simulink model "SatelliteAttitudeTargeting"  (R2020b)
settings: Solver=VariableStepAuto  StartTime=0.0  StopTime=30  MinStep=5e-5  RelTol=2.8421709430404007E-14
values from neighbouring files (symbols this model uses):
  dt_delay = 0.01    [main.m]
  hwdotmax = 0.004    [controlDesign.m]
  hwmax = 0.015    [controlDesign.m]
  Kd = diag([Kd1; Kd2; Kd3])    [controlDesign.m]
  Ko = 3075    [controlDesign.m]
  Kp = 8.0    (= 8)    [controlDesign.m]
  Po = 400    [controlDesign.m]
  s = tf('s')    [controlDesign.m]
  safety = 0.5    [controlDesign.m]
  wn = 2*pi*10    (= 62.8318530718)    [controlDesign.m]
  zeta = sqrt(2)/2    [controlDesign.m]
  Zo = 0.01    [controlDesign.m]
undefined symbols (not defined in the file or in its folder): A_BP, A_PB, J_C_B, J_C_P, md, ms, q_PB, rcb_B, rlb_B, X, Y, Z
libraries: sm_lib x10, nesl_utility x4
settings Model: Creator=bbingham  LastModifiedBy=tjones
settings SolverCC: MaxConsecutiveMinStep=2
settings DataIOCC: SaveOutput=off  SignalLogging=off  DSMLogging=off  ReturnWorkspaceOutputs=off
settings DebuggingCC: ArithmeticOperatorsInVariantConditions=warning
settings SFSimCC: SimUseLocalCustomCode=off  CustomCodeUndefinedFunction=UseInterfaceOnly
settings RTWCC: Description=Simulink Desktop Real-Time  SystemTargetFile=sldrt.tlc  TemplateMakefile=sldrt.tmf  RTWUseLocalCustomCode=off  RTWCompilerOptimization=on
settings CodeAppCC: MaxIdLength=95  StateflowObjectComments=on
settings TargetCC: TargetPreCompLibLocation=C:\Program Files\MATLAB\R2020a\toolbox\sldrt\lib\win64  TargetLangStandard=C99 (ISO)  SupportVariableSizeSignals=on
settings SimscapeCC: SimscapeNormalizeSystem=off

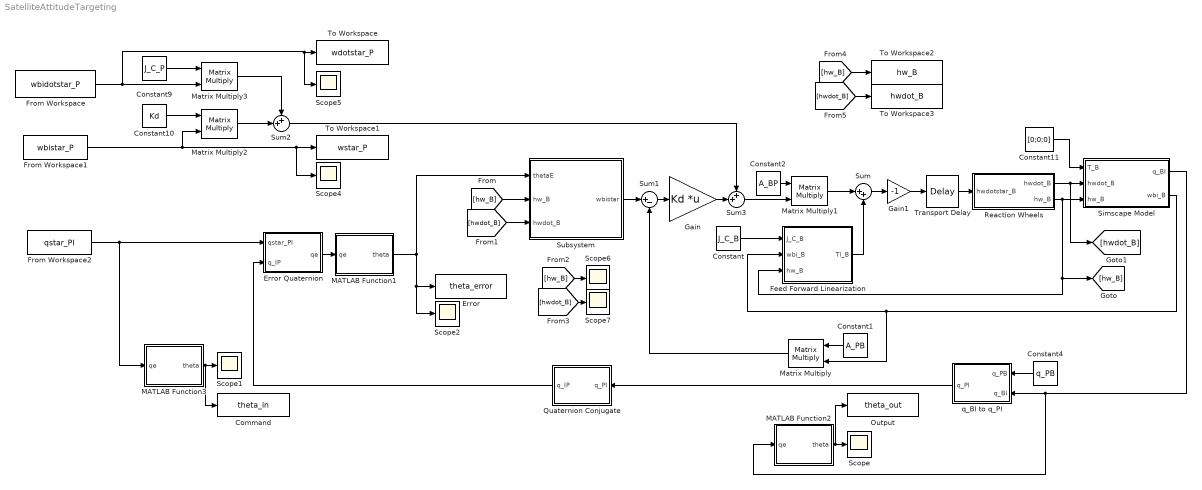
== system SatelliteAttitudeTargeting ==
  Command : ToWorkspace  VariableName=theta_in  SaveFormat=Timeseries  SampleTime=-1
  Constant : Constant  Value=J_C_B
  Constant1 : Constant  Value=A_PB
  Constant10 : Constant  Value=Kd
  Constant11 : Constant  Value=[0;0;0]
  Constant2 : Constant  Value=A_BP
  Constant4 : Constant  Value=q_PB  OutDataTypeStr=Bus: qBus
  Constant9 : Constant  Value=J_C_P
  Error : ToWorkspace  VariableName=theta_error  SaveFormat=Timeseries  SampleTime=-1
  Error Quaternion : MATLAB Function  TreatAsAtomicUnit=on
  Feed Forward Linearization : MATLAB Function  TreatAsAtomicUnit=on
  From Workspace : FromWorkspace  VariableName=wbidotstar_P
  From Workspace1 : FromWorkspace  VariableName=wbistar_P
  From Workspace2 : FromWorkspace  VariableName=qstar_PI  OutDataTypeStr=Bus: qBus
  Gain : Gain  Gain=Kd  Multiplication=Matrix(K*u) (u vector)
  Gain1 : Gain  Gain=-1
  MATLAB Function1 : MATLAB Function  TreatAsAtomicUnit=on
  MATLAB Function2 : MATLAB Function  TreatAsAtomicUnit=on
  MATLAB Function3 : MATLAB Function  TreatAsAtomicUnit=on
  Matrix Multiply{,1..3} (4 alike) : Product  Multiplication=Matrix(*)
  Output : ToWorkspace  VariableName=theta_out  SaveFormat=Timeseries  SampleTime=-1
  Quaternion Conjugate : MATLAB Function  TreatAsAtomicUnit=on
  Reaction Wheels : Subsystem
  Scope{,1..2,4..7} (7 alike) : Scope
  Simscape Model : Subsystem  TreatAsAtomicUnit=on
  Subsystem : Subsystem
  Sum : Sum  Inputs=|++
  Sum1 : Sum  Inputs=|+-
  Sum2 : Sum  Inputs=++|
  Sum3 : Sum  Inputs=++|
  To Workspace : ToWorkspace  VariableName=wdotstar_P  SaveFormat=Timeseries  SampleTime=-1
  To Workspace1 : ToWorkspace  VariableName=wstar_P  SaveFormat=Timeseries  SampleTime=-1
  To Workspace2 : ToWorkspace  VariableName=hw_B  SaveFormat=Timeseries  SampleTime=-1
  To Workspace3 : ToWorkspace  VariableName=hwdot_B  SaveFormat=Timeseries  SampleTime=-1
  Transport Delay : TransportDelay  DelayTime=dt_delay  BufferSize=3072
  q_BI to q_PI : MATLAB Function  TreatAsAtomicUnit=on
  wires:
  Simscape Model/2(wbi_B) -> Matrix Multiply/2, Feed Forward Linearization/2(wbi_B)
  Feed Forward Linearization/1(Tl_B) -> Sum/2
  Constant/1 -> Feed Forward Linearization/1(J_C_B)
  Constant1/1 -> Matrix Multiply/1
  Matrix Multiply/1 -> Sum1/2
  Sum1/1 -> Gain/1
  Constant2/1 -> Matrix Multiply1/1
  Matrix Multiply1/1 -> Sum/1
  Constant4/1 -> q_BI to q_PI/1(q_PB)
  Simscape Model/1(q_BI) -> MATLAB Function2/1(qe), q_BI to q_PI/2(q_BI)
  q_BI to q_PI/1(q_PI) -> Quaternion Conjugate/1(q_PI)
  Error Quaternion/1(qe) -> MATLAB Function1/1(qe)
  From Workspace2/1 -> Error Quaternion/1(qstar_PI), MATLAB Function3/1(qe)
  Quaternion Conjugate/1(q_IP) -> Error Quaternion/2(q_IP)
  MATLAB Function1/1(theta) -> Subsystem/1(thetaE), Error/1, Scope2/1
  MATLAB Function2/1(theta) -> Output/1, Scope/1
  MATLAB Function3/1(theta) -> Command/1, Scope1/1
  Sum/1 -> Gain1/1
  Gain1/1 -> Transport Delay/1
  Transport Delay/1 -> Reaction Wheels/1(hwdotstar_B)
  Reaction Wheels/2(hw_B) -> Simscape Model/3(hw_B), Feed Forward Linearization/3(hw_B), [hw_B]
  Reaction Wheels/1(hwdot_B) -> [hwdot_B], Simscape Model/2(hwdot_B)
  Subsystem/1(wbistar) -> Sum1/1
  [hw_B] -> Subsystem/2(hw_B)
  [hwdot_B] -> Subsystem/3(hwdot_B)
  Constant9/1 -> Matrix Multiply3/1
  Constant10/1 -> Matrix Multiply2/1
  Matrix Multiply3/1 -> Sum2/1
  Matrix Multiply2/1 -> Sum2/2
  Gain/1 -> Sum3/2
  Sum2/1 -> Sum3/1
  Sum3/1 -> Matrix Multiply1/2
  From Workspace1/1 -> Matrix Multiply2/2, Scope4/1, To Workspace1/1
  From Workspace/1 -> Scope5/1, To Workspace/1, Matrix Multiply3/2
  [hw_B] -> Scope6/1
  [hwdot_B] -> Scope7/1
  [hw_B] -> To Workspace2/1
  [hwdot_B] -> To Workspace3/1
  Constant11/1 -> Simscape Model/1(T_B)

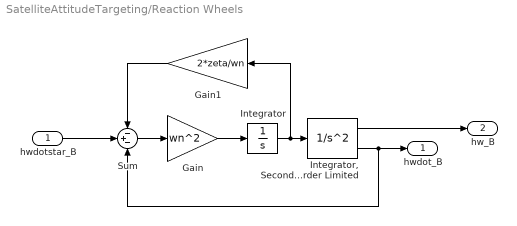
== system SatelliteAttitudeTargeting/Reaction Wheels ==
  hwdotstar_B : Inport
  Gain : Gain  Gain=wn^2
  Gain1 : Gain  Gain=2*zeta/wn
  Integrator : Integrator
  "Integrator, Second-Order Limited" : SecondOrderIntegrator  ICX=hw0_B  LimitX=on  UpperLimitX=hwmax  LowerLimitX=-hwmax  LimitDXDT=on  UpperLimitDXDT=hwdotmax  LowerLimitDXDT=-hwdotmax
  Sum : Sum  Inputs=-+-
  hwdot_B : Outport
  hw_B : Outport  Port=2
  wires:
  Sum/1 -> Gain/1
  Gain/1 -> Integrator/1
  Integrator/1 -> Gain1/1, "Integrator, Second-Order Limited"/1
  "Integrator, Second-Order Limited"/2 -> Sum/3, hwdot_B/1
  "Integrator, Second-Order Limited"/1 -> hw_B/1
  hwdotstar_B/1 -> Sum/2
  Gain1/1 -> Sum/1

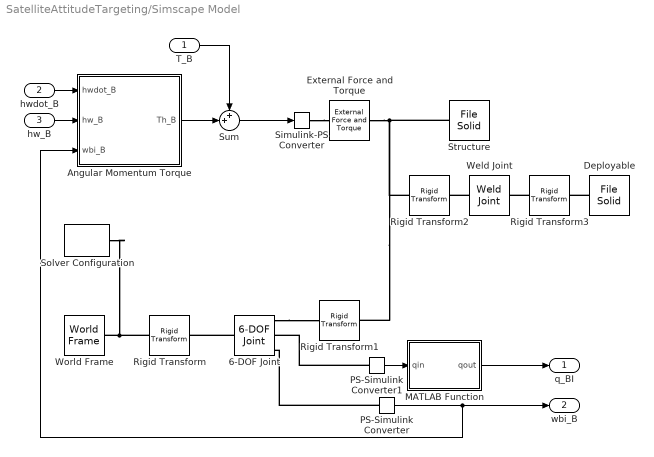
== system SatelliteAttitudeTargeting/Simscape Model ==
  T_B : Inport
  hwdot_B : Inport  Port=2
  hw_B : Inport  Port=3
  6-DOF Joint : sm_lib/Joints/6-DOF Joint  JointMode=Normal  SenseConstraintForce=off  SenseConstraintForceX=off  SenseConstraintForceY=off  SenseConstraintForceZ=off  SenseConstraintTorque=off  SenseConstraintTorqueX=off  SenseConstraintTorqueY=off  SenseConstraintTorqueZ=off  SenseTotalForce=off  SenseTotalForceX=off  SenseTotalForceY=off  SenseTotalForceZ=off  SenseTotalTorque=off  SenseTotalTorqueX=off  SenseTotalTorqueY=off  SenseTotalTorqueZ=off  CompositeWrenchDir=FollowerOnBase  CompositeWrenchFrame=BaseFrame  PxEquilibriumPosition=0  PxEquilibriumPositionUnits=m  PxSpringStiffness=0  PxSpringStiffnessUnits=N/m  PxDampingCoefficient=0  PxDampingCoefficientUnits=N/(m/s)  PxTorqueActuationMode=NoTorque  PxMotionActuationMode=ComputedMotion  PxSensePosition=off  PxSenseVelocity=off  PxSenseAcceleration=off  PxSenseTorqueForce=off  PxSenseLowerLimitTorqueForce=off  PxSenseUpperLimitTorqueForce=off  PxLowerLimitSpecify=off  PxLowerLimitBound=-1  PxLowerLimitBoundUnits=m  PxLowerLimitStiffness=1e6  PxLowerLimitStiffnessUnits=N/m  PxLowerLimitDamping=1e3  PxLowerLimitDampingUnits=N/(m/s)  PxLowerLimitTransitionRegionWidth=1e-4  PxLowerLimitTransitionRegionWidthUnits=m  PxUpperLimitSpecify=off  PxUpperLimitBound=1  PxUpperLimitBoundUnits=m  PxUpperLimitStiffness=1e6  PxUpperLimitStiffnessUnits=N/m  PxUpperLimitDamping=1e3  PxUpperLimitDampingUnits=N/(m/s)  PxUpperLimitTransitionRegionWidth=1e-4  PxUpperLimitTransitionRegionWidthUnits=m  PxPositionTargetSpecify=off  PxPositionTargetPriority=High  PxPositionTargetValue=0  PxPositionTargetValueUnits=m  PxVelocityTargetSpecify=off  PxVelocityTargetPriority=High  PxVelocityTargetValue=0  PxVelocityTargetValueUnits=m/s  PyEquilibriumPosition=0  PyEquilibriumPositionUnits=m  PySpringStiffness=0  PySpringStiffnessUnits=N/m  PyDampingCoefficient=0  PyDampingCoefficientUnits=N/(m/s)  PyTorqueActuationMode=NoTorque  PyMotionActuationMode=ComputedMotion  PySensePosition=off  PySenseVelocity=off  PySenseAcceleration=off  PySenseTorqueForce=off  PySenseLowerLimitTorqueForce=off  PySenseUpperLimitTorqueForce=off  PyLowerLimitSpecify=off  PyLowerLimitBound=-1  PyLowerLimitBoundUnits=m  PyLowerLimitStiffness=1e6  PyLowerLimitStiffnessUnits=N/m  PyLowerLimitDamping=1e3  PyLowerLimitDampingUnits=N/(m/s)  PyLowerLimitTransitionRegionWidth=1e-4  PyLowerLimitTransitionRegionWidthUnits=m  PyUpperLimitSpecify=off  PyUpperLimitBound=1  PyUpperLimitBoundUnits=m  PyUpperLimitStiffness=1e6  PyUpperLimitStiffnessUnits=N/m  PyUpperLimitDamping=1e3  PyUpperLimitDampingUnits=N/(m/s)  PyUpperLimitTransitionRegionWidth=1e-4  PyUpperLimitTransitionRegionWidthUnits=m  PyPositionTargetSpecify=off  PyPositionTargetPriority=High  PyPositionTargetValue=0  PyPositionTargetValueUnits=m  PyVelocityTargetSpecify=off  PyVelocityTargetPriority=High  PyVelocityTargetValue=0  PyVelocityTargetValueUnits=m/s  PzEquilibriumPosition=0  PzEquilibriumPositionUnits=m  PzSpringStiffness=0  PzSpringStiffnessUnits=N/m  PzDampingCoefficient=0  PzDampingCoefficientUnits=N/(m/s)  PzTorqueActuationMode=NoTorque  PzMotionActuationMode=ComputedMotion  PzSensePosition=off  PzSenseVelocity=off  PzSenseAcceleration=off  PzSenseTorqueForce=off  PzSenseLowerLimitTorqueForce=off  PzSenseUpperLimitTorqueForce=off  PzLowerLimitSpecify=off  PzLowerLimitBound=-1  PzLowerLimitBoundUnits=m  PzLowerLimitStiffness=1e6  PzLowerLimitStiffnessUnits=N/m  PzLowerLimitDamping=1e3  PzLowerLimitDampingUnits=N/(m/s)  PzLowerLimitTransitionRegionWidth=1e-4  PzLowerLimitTransitionRegionWidthUnits=m  PzUpperLimitSpecify=off  PzUpperLimitBound=1  PzUpperLimitBoundUnits=m  PzUpperLimitStiffness=1e6  PzUpperLimitStiffnessUnits=N/m  PzUpperLimitDamping=1e3  PzUpperLimitDampingUnits=N/(m/s)  PzUpperLimitTransitionRegionWidth=1e-4  PzUpperLimitTransitionRegionWidthUnits=m  PzPositionTargetSpecify=off  PzPositionTargetPriority=High  PzPositionTargetValue=0  PzPositionTargetValueUnits=m  PzVelocityTargetSpecify=off  PzVelocityTargetPriority=High  PzVelocityTargetValue=0  PzVelocityTargetValueUnits=m/s  SphDefPosRotationMethod=None  SphDefPosRotationAngleUnits=deg  SphDefPosRotationStandardAxis=+Z  SphDefPosRotationAngle=0.0  SphDefPosRotationArbitraryAxis=[0 0 1]  SphDefPosFollAlignAxisA=+X  SphDefPosBaseAlignAxisA=+Y  SphDefPosFollAlignAxisB=+Y  SphDefPosBaseAlignAxisB=+Z  SphDefPosRotationSequenceAxes=FollowerAxes  SphDefPosRotationSequence=XYX  SphDefPosRotationSequenceAngles=[0 0 0]  SphDefPosRotationSequenceAnglesUnits=deg  SphDefPosRotationMatrix=[1 0 0; 0 1 0; 0 0 1]  SphEqPosRotationMethod=None  SphEqPosRotationAngleUnits=deg  SphEqPosRotationStandardAxis=+Z  SphEqPosRotationAngle=0.0  SphEqPosRotationArbitraryAxis=[0 0 1]  SphEqPosFollAlignAxisA=+X  SphEqPosBaseAlignAxisA=+Y  SphEqPosFollAlignAxisB=+Y  SphEqPosBaseAlignAxisB=+Z  SphEqPosRotationSequenceAxes=FollowerAxes  SphEqPosRotationSequence=XYX  SphEqPosRotationSequenceAngles=[0 0 0]  SphEqPosRotationSequenceAnglesUnits=deg  SphEqPosRotationMatrix=[1 0 0; 0 1 0; 0 0 1]  SphSpringStiffness=0  SphSpringStiffnessUnits=N*m/deg  SphDampingCoefficient=0  SphDampingCoefficientUnits=N*m/(deg/s)  SphActuateTorqueX=off  SphActuateTorqueY=off  SphActuateTorqueZ=off  SphActuateTorque=off  SphTorqueActuationMode=NoTorque  SphMotionActuationMode=ComputedMotion  SphActuationFrame=BaseFrame  SphSensePosition=on  SphSenseVelocityX=off  SphSenseVelocityY=off  SphSenseVelocityZ=off  SphSenseVelocity=on  SphSenseAccelerationX=off  SphSenseAccelerationY=off  SphSenseAccelerationZ=off  SphSenseAcceleration=off  SphSenseTorqueX=off  SphSenseTorqueY=off  SphSenseTorqueZ=off  SphSenseTorqueForce=off  SphSenseLowerLimitTorqueMag=off  SphSenseUpperLimitTorqueMag=off  SphSensingFrame=FollowerFrame  SphLowerLimitSpecify=off  SphLowerLimitBound=15  SphLowerLimitBoundUnits=deg  SphLowerLimitStiffness=1e4  SphLowerLimitStiffnessUnits=N*m/deg  SphLowerLimitDamping=10  SphLowerLimitDampingUnits=N*m/(deg/s)  SphLowerLimitTransitionRegionWidth=0.1  SphLowerLimitTransitionRegionWidthUnits=deg  SphUpperLimitSpecify=off  SphUpperLimitBound=45  SphUpperLimitBoundUnits=deg  SphUpperLimitStiffness=1e4  SphUpperLimitStiffnessUnits=N*m/deg  SphUpperLimitDamping=10  SphUpperLimitDampingUnits=N*m/(deg/s)  SphUpperLimitTransitionRegionWidth=0.1  SphUpperLimitTransitionRegionWidthUnits=deg  SphPositionTargetRotationMethod=RotationMatrix  SphPositionTargetRotationAngleUnits=deg  SphPositionTargetRotationStandardAxis=+Z  SphPositionTargetRotationAngle=0.0  SphPositionTargetRotationArbitraryAxis=[0 0 1]  SphPositionTargetFollAlignAxisA=+X  SphPositionTargetBaseAlignAxisA=+Y  SphPositionTargetFollAlignAxisB=+Y  SphPositionTargetBaseAlignAxisB=+Z  SphPositionTargetRotationSequenceAxes=FollowerAxes  SphPositionTargetRotationSequence=XYX  SphPositionTargetRotationSequenceAngles=[0 0 0]  SphPositionTargetRotationSequenceAnglesUnits=deg  SphPositionTargetRotationMatrix=A0_IB  SphPositionTargetSpecify=on  SphPositionTargetPriority=High  SphVelocityTargetValue=wbi0_B  SphVelocityTargetValueUnits=rad/s  SphVelocityTargetSpecify=on  SphVelocityTargetPriority=High  SphVelocityTargetInFollowerFrame=on
  Angular Momentum Torque : MATLAB Function  TreatAsAtomicUnit=on
  Deployable : sm_lib/Body Elements/File Solid  ExtGeomFileName=/home/tjones/Documents/School/SpacecraftAttitudeControl/03 Attitude Dynamics/deployable.STL  UnitType=Custom  ExtGeomFileUnits=mm  StepReaderType=HEX  ExportConvexHullGeometry=off  InertiaType=Custom  Mass=md  MassUnits=kg  CenterOfMass=rdb_B  CenterOfMassUnits=m  MomentsOfInertia=Md_D_B  MomentsOfInertiaUnits=kg*m^2  ProductsOfInertia=Pd_D_B  ProductsOfInertiaUnits=kg*m^2  BasedOnType=DensityFromFile  Density=1000  DensityUnits=kg/m^3  DoExposeReferenceFrame=on  SerializedFrames=<Frames/>  GraphicType=FromGeometry  MarkerShape=Sphere  MarkerSize=10  GraphicVisPropType=SimpleVisualProperties  GraphicDiffuseColor=[1.0 0.6 0.4]  GraphicSpecularColor=[0.5 0.5 0.5 1.0]  GraphicAmbientColor=[0.15 0.15 0.15 1.0]  GraphicEmissiveColor=[0.0 0.0 0.0 1.0]  GraphicShininess=75  GraphicOpacity=1.0
  External Force and Torque : sm_lib/Forces and Torques/External Force and Torque  ForceResolutionFrame=AttachedFrame  EnableForceX=off  EnableForceY=off  EnableForceZ=off  EnableForce=off  TorqueResolutionFrame=AttachedFrame  EnableTorqueX=off  EnableTorqueY=off  EnableTorqueZ=off  EnableTorque=on
  MATLAB Function : MATLAB Function  TreatAsAtomicUnit=on
  PS-Simulink Converter : nesl_utility/PS-Simulink Converter  PhysicalDomain=network_engine_domain  SubClassName=ps_output  LeftPortType=input  RightPortType=output  PseudoPeriodic=off  Frequencies=[]  Unit=inherit  AffineConversion=off
  PS-Simulink Converter1 : nesl_utility/PS-Simulink Converter  PhysicalDomain=network_engine_domain  SubClassName=ps_output  LeftPortType=input  RightPortType=output  PseudoPeriodic=off  Frequencies=[]  Unit=inherit  AffineConversion=off
  Rigid Transform : sm_lib/Frames and Transforms/Rigid Transform  TranslationMethod=Cartesian  TranslationStandardOffset=0  TranslationLengthUnit=m  TranslationStandardAxis=+Z  TranslationCartesianOffset=rcb_B  TranslationROffset=0  TranslationROffsetUnits=m  TranslationZOffset=0  TranslationZOffsetUnits=m  TranslationThetaOffset=0  TranslationThetaOffsetUnits=deg  RotationMethod=None  RotationAngleUnits=deg  RotationStandardAxis=+Z  RotationAngle=0.0  RotationArbitraryAxis=[0 0 1]  FollAlignAxisA=+X  BaseAlignAxisA=+Y  FollAlignAxisB=+Y  BaseAlignAxisB=+Z  RotationSequenceAxes=FollowerAxes  RotationSequence=XYX  RotationSequenceAngles=[0 0 0]  RotationSequenceAnglesUnits=deg  RotationMatrix=[1 0 0; 0 1 0; 0 0 1]
  Rigid Transform1 : sm_lib/Frames and Transforms/Rigid Transform  TranslationMethod=Cartesian  TranslationStandardOffset=0  TranslationLengthUnit=m  TranslationStandardAxis=+Z  TranslationCartesianOffset=-rcb_B  TranslationROffset=0  TranslationROffsetUnits=m  TranslationZOffset=0  TranslationZOffsetUnits=m  TranslationThetaOffset=0  TranslationThetaOffsetUnits=deg  RotationMethod=None  RotationAngleUnits=deg  RotationStandardAxis=+Z  RotationAngle=0.0  RotationArbitraryAxis=[0 0 1]  FollAlignAxisA=+X  BaseAlignAxisA=+Y  FollAlignAxisB=+Y  BaseAlignAxisB=+Z  RotationSequenceAxes=FollowerAxes  RotationSequence=XYX  RotationSequenceAngles=[0 0 0]  RotationSequenceAnglesUnits=deg  RotationMatrix=[1 0 0; 0 1 0; 0 0 1]
  Rigid Transform2 : sm_lib/Frames and Transforms/Rigid Transform  TranslationMethod=Cartesian  TranslationStandardOffset=0  TranslationLengthUnit=m  TranslationStandardAxis=+Z  TranslationCartesianOffset=rlb_B  TranslationROffset=0  TranslationROffsetUnits=m  TranslationZOffset=0  TranslationZOffsetUnits=m  TranslationThetaOffset=0  TranslationThetaOffsetUnits=deg  RotationMethod=None  RotationAngleUnits=deg  RotationStandardAxis=+Z  RotationAngle=0.0  RotationArbitraryAxis=[0 0 1]  FollAlignAxisA=+X  BaseAlignAxisA=+Y  FollAlignAxisB=+Y  BaseAlignAxisB=+Z  RotationSequenceAxes=FollowerAxes  RotationSequence=XYX  RotationSequenceAngles=[0 0 0]  RotationSequenceAnglesUnits=deg  RotationMatrix=[1 0 0; 0 1 0; 0 0 1]
  Rigid Transform3 : sm_lib/Frames and Transforms/Rigid Transform  TranslationMethod=Cartesian  TranslationStandardOffset=0  TranslationLengthUnit=m  TranslationStandardAxis=+Z  TranslationCartesianOffset=-rlb_B  TranslationROffset=0  TranslationROffsetUnits=m  TranslationZOffset=0  TranslationZOffsetUnits=m  TranslationThetaOffset=0  TranslationThetaOffsetUnits=deg  RotationMethod=None  RotationAngleUnits=deg  RotationStandardAxis=+Z  RotationAngle=0.0  RotationArbitraryAxis=[0 0 1]  FollAlignAxisA=+X  BaseAlignAxisA=+Y  FollAlignAxisB=+Y  BaseAlignAxisB=+Z  RotationSequenceAxes=FollowerAxes  RotationSequence=XYX  RotationSequenceAngles=[0 0 0]  RotationSequenceAnglesUnits=deg  RotationMatrix=[1 0 0; 0 1 0; 0 0 1]
  Simulink-PS Converter : nesl_utility/Simulink-PS Converter  PhysicalDomain=network_engine_domain  SubClassName=ps_input  LeftPortType=input  RightPortType=output  PseudoPeriodic=off  Frequencies=[]  NoiseDistribution=none  NoiseParameters=[]  Unit=1  AffineConversion=off  FilteringAndDerivatives=provide  SimscapeFilterOrder=1  InputFilterTimeConstant=0.001  UdotUserProvided=0
  Solver Configuration : nesl_utility/Solver Configuration  PhysicalDomain=network_engine_domain  SubClassName=solver  LeftPortType=input  RightPortType=generic  Tones=[]  Harmonics=[]  SimulateNoise=off  Profile=off  UseLocalSampling=off  EnableSwitchedLinearOptims=on  FrequencyDomain=off  UseCCode=off  RelTol=0.001  AbsTol=1e-06  MinStep=1e-09  ToWorkspace=off  RevertToSquareIcSolve=off  NumHomotopyIterations=100  PhasorMode=off  PhasorModeNumHarmonics=1  DoDC=off  ResidualTolerance=1e-12  UseLocalSolver=off  LocalSolverChoice=NE_BACKWARD_EULER_ADVANCER  LocalSolverSampleTime=0.001  DoFixedCost=off  MaxNonlinIter=3  MaxModeIter=2  ComputeImpulses=off  ImpulseIterations=2  LinearAlgebra=auto  EquationFormulation=NE_TIME_EF  DelaysMemoryBudget=1024  AutomaticFiltering=on  FilteringTimeConstant=0.001  PartitionStorageMethod=AS_NEEDED  PartitionMemoryBudget=1024  PartitionMethod=ROBUST
  Structure : sm_lib/Body Elements/File Solid  ExtGeomFileName=/home/tjones/Documents/School/SpacecraftAttitudeControl/03 Attitude Dynamics/structure.STL  UnitType=Custom  ExtGeomFileUnits=mm  StepReaderType=HEX  ExportConvexHullGeometry=off  InertiaType=Custom  Mass=ms  MassUnits=kg  CenterOfMass=rsb_B  CenterOfMassUnits=m  MomentsOfInertia=Ms_S_B  MomentsOfInertiaUnits=kg*m^2  ProductsOfInertia=Ps_S_B  ProductsOfInertiaUnits=kg*m^2  BasedOnType=DensityFromFile  Density=1000  DensityUnits=kg/m^3  DoExposeReferenceFrame=on  SerializedFrames=<Frames/>  GraphicType=FromGeometry  MarkerShape=Sphere  MarkerSize=10  GraphicVisPropType=SimpleVisualProperties  GraphicDiffuseColor=[0.6 1.0 0.6]  GraphicSpecularColor=[0.5 0.5 0.5 1.0]  GraphicAmbientColor=[0.15 0.15 0.15 1.0]  GraphicEmissiveColor=[0.0 0.0 0.0 1.0]  GraphicShininess=75  GraphicOpacity=1.0
  Sum : Sum  Inputs=++|
  Weld Joint : sm_lib/Joints/Weld Joint  JointMode=Normal  SenseConstraintForce=off  SenseConstraintForceX=off  SenseConstraintForceY=off  SenseConstraintForceZ=off  SenseConstraintTorque=off  SenseConstraintTorqueX=off  SenseConstraintTorqueY=off  SenseConstraintTorqueZ=off  SenseTotalForce=off  SenseTotalForceX=off  SenseTotalForceY=off  SenseTotalForceZ=off  SenseTotalTorque=off  SenseTotalTorqueX=off  SenseTotalTorqueY=off  SenseTotalTorqueZ=off  CompositeWrenchDir=FollowerOnBase  CompositeWrenchFrame=BaseFrame
  World Frame : sm_lib/Frames and Transforms/World Frame
  q_BI : Outport  OutDataTypeStr=Bus: qBus  VectorParamsAs1DForOutWhenUnconnected=off
  wbi_B : Outport  Port=2  VectorParamsAs1DForOutWhenUnconnected=off
  wires:
  MATLAB Function/1(qout) -> q_BI/1
  PS-Simulink Converter1/1 -> MATLAB Function/1(qin)
  PS-Simulink Converter/1 -> Angular Momentum Torque/3(wbi_B), wbi_B/1
  Angular Momentum Torque/1(Th_B) -> Sum/2
  hwdot_B/1 -> Angular Momentum Torque/1(hwdot_B)
  hw_B/1 -> Angular Momentum Torque/2(hw_B)
  T_B/1 -> Sum/1
  Sum/1 -> Simulink-PS Converter/1
  connections:
  World Frame/RConn1 -- Solver Configuration/RConn1 -- Rigid Transform/LConn1
  External Force and Torque/RConn1 -- Structure/RConn1 -- Rigid Transform2/LConn1 -- Rigid Transform1/RConn1
  Simulink-PS Converter/RConn1 -- External Force and Torque/LConn1
  Deployable/RConn1 -- Rigid Transform3/RConn1
  Weld Joint/LConn1 -- Rigid Transform2/RConn1
  6-DOF Joint/LConn1 -- Rigid Transform/RConn1
  PS-Simulink Converter1/LConn1 -- 6-DOF Joint/RConn2
  6-DOF Joint/RConn1 -- Rigid Transform1/LConn1
  PS-Simulink Converter/LConn1 -- 6-DOF Joint/RConn3
  Rigid Transform3/LConn1 -- Weld Joint/RConn1

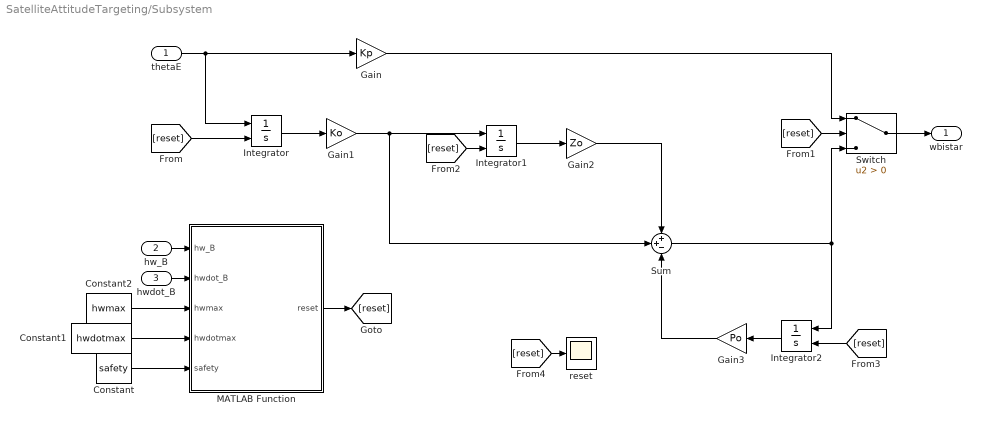
== system SatelliteAttitudeTargeting/Subsystem ==
  thetaE : Inport
  hw_B : Inport  Port=2
  hwdot_B : Inport  Port=3
  Constant : Constant  Value=safety
  Constant1 : Constant  Value=hwdotmax
  Constant2 : Constant  Value=hwmax
  Gain : Gain  Gain=Kp
  Gain1 : Gain  Gain=Ko
  Gain2 : Gain  Gain=Zo
  Gain3 : Gain  Gain=Po
  Integrator : Integrator  ExternalReset=level
  Integrator1 : Integrator  ExternalReset=level
  Integrator2 : Integrator  ExternalReset=level
  MATLAB Function : MATLAB Function  TreatAsAtomicUnit=on
  Sum : Sum  Inputs=++-
  Switch : Switch  Criteria=u2 > Threshold
  reset : Scope
  wbistar : Outport
  wires:
  thetaE/1 -> Integrator/1, Gain/1
  Constant/1 -> MATLAB Function/5(safety)
  Constant1/1 -> MATLAB Function/4(hwdotmax)
  Constant2/1 -> MATLAB Function/3(hwmax)
  hw_B/1 -> MATLAB Function/1(hw_B)
  hwdot_B/1 -> MATLAB Function/2(hwdot_B)
  Switch/1 -> wbistar/1
  Gain/1 -> Switch/1
  MATLAB Function/1(reset) -> [reset]
  [reset] -> Integrator/2
  [reset] -> Switch/2
  Integrator/1 -> Gain1/1
  Gain1/1 -> Sum/2, Integrator1/1
  [reset] -> Integrator1/2
  Integrator1/1 -> Gain2/1
  Gain2/1 -> Sum/1
  Sum/1 -> Integrator2/1, Switch/3
  [reset] -> Integrator2/2
  Integrator2/1 -> Gain3/1
  Gain3/1 -> Sum/3
  [reset] -> reset/1

== matlab function SatelliteAttitudeTargeting/Simscape Model/MATLAB Function ==
  data: qin input; qout output Bus: qBus
function qout = fcn(qin)

qout.s = qin(1);
qout.v = qin(2:4);

== matlab function SatelliteAttitudeTargeting/Feed Forward Linearization ==
  data: J_C_B input; Tl_B output; wbi_B input; hw_B input
function Tl_B = fcn(J_C_B, wbi_B, hw_B)

Tl_B = cross(wbi_B, J_C_B*wbi_B + hw_B);

== matlab function SatelliteAttitudeTargeting/MATLAB Function2 ==
  data: qe input; theta output
function theta = fcn(qe)

qe = qUnit(qe);

[e, angle] = q2e(qe);

theta = e*angle;

== matlab function SatelliteAttitudeTargeting/q_BI to q_PI ==
  data: q_PB input; q_PI output Bus: qBus; q_BI input
function q_PI = fcn(q_PB, q_BI)

q_PI = qX(q_PB, q_BI);

== matlab function SatelliteAttitudeTargeting/Quaternion Conjugate ==
  data: q_PI input Bus: qBus; q_IP output Bus: qBus
function q_IP = fcn(q_PI)

q_IP = qT(q_PI);

== matlab function SatelliteAttitudeTargeting/Error Quaternion ==
  data: qstar_PI input Bus: qBus; qe output Bus: qBus; q_IP input Bus: qBus
function qe = fcn(qstar_PI, q_IP)

qe = qX(qstar_PI, q_IP);

== matlab function SatelliteAttitudeTargeting/MATLAB Function1 ==
  data: qe input; theta output
function theta = fcn(qe)

qe = qUnit(qe);

[e, angle] = q2e(qe);

theta = e*angle;

== matlab function SatelliteAttitudeTargeting/MATLAB Function3 ==
  data: qe input Bus: qBus; theta output
function theta = fcn(qe)

qe = qUnit(qe);

[e, angle] = q2e(qe);

theta = e*angle;

== matlab function SatelliteAttitudeTargeting/Simscape Model/Angular Momentum Torque ==
  data: hwdot_B input; Th_B output; hw_B input; wbi_B input
function Th_B = fcn(hwdot_B, hw_B, wbi_B)

Th_B = -hwdot_B - cross(wbi_B, hw_B);

== matlab function SatelliteAttitudeTargeting/Subsystem/MATLAB Function ==
  data: hw_B input; reset output; hwdot_B input; hwmax input; hwdotmax input; safety input
function reset = fcn(hw_B, hwdot_B, hwmax, hwdotmax, safety)

reset = 0;
if(max(abs(hw_B)) > (hwmax * safety) || ...
    max(abs(hwdot_B)) > (hwdotmax * safety))
  reset = 1;
end
